simulink model "bh_model_crank_dynamics"  (R2022b)
settings: Solver=ode15s  StartTime=0.0  StopTime=45  RelTol=1e-4  AbsTol=1e-4  EnableMultiTasking=on
undefined symbols (not defined in the file): IC, params, sigbuilder_block, X, Y, Z
libraries: sm_lib x21, nesl_utility x19, simulink_extras x11, simulink x2
(part 1 of 2)
settings Model: Creator=bhorton  LastModifiedBy=bhorton
settings SolverCC: AutoScaleAbsTol=off  ZeroCrossAlgorithm=Adaptive  AlgebraicLoopSolver=TrustRegion
settings DataIOCC: LimitDataPoints=on  MaxDataPoints=10000
settings OptimizationCC: LifeSpan=inf
settings DebuggingCC: UnconnectedInputMsg=warning  UnconnectedOutputMsg=warning  UnconnectedLineMsg=warning  AllowSymbolicDim=off  SFUnexpectedBacktrackingDiag=warning  SFNoUnconditionalDefaultTransitionDiag=warning  SFExecutionAtInitializationDiag=none  SFMachineParentedDataDiag=warning  ArithmeticOperatorsInVariantConditions=warning
settings ModelReferenceCC: EnableRefExpFcnMdlSchedulingChecks=on
settings SFSimCC: SimUseLocalCustomCode=off  CustomCodeUndefinedFunction=UseInterfaceOnly
settings RTWCC: RTWUseLocalCustomCode=off  DLArmComputeVersion=19.05
settings CodeAppCC: StateflowObjectComments=on
settings GRTTargetCC: TargetLangStandard=C89/C90 (ANSI)
settings ConfigComp: CovMetricSettings=dw  CovSaveCumulativeToWorkspaceVar=on  CovSaveSingleToWorkspaceVar=on  CovExternalEMLEnable=off  CovSFcnEnable=off
settings SimscapeCC: SimscapeLogType=all  SimscapeLogSimulationStatistics=on  SimscapeLogToSDI=on  SimscapeLogLimitData=off  SimscapeLogDataHistory=10000
settings ExplorerConfigSet: InternalSimMechanicsExplorerSettings="<ExplorerConfiguration><canonicalview>default</canonicalview><AnimationSetting><BasePlaybackSpeed>1.0</BasePlaybackSpeed><PlaybackSpeedFactor>1.0</PlaybackSpeedFactor></AnimationSetting><TilePanel><TileInfo><Tiles Columns=\"1\" Count=\"1\" Rows=\"1\"><Column Weight=\"1\"/><Row Weight=\"1\"/><Tile Height=\"1\" Width=\"1\" X=\"0\" Y=\"0\"/></Tiles></TileInfo><SceneInfo><SceneViewer><BGColor><R>0.60000002384185791</R><G>0.60000002384185791</G><B>0.60000002384185791</B></BGColor><Camera><DoPerspective>off</DoPerspective><Position><X>0.384574720736644893</X><Y>0.1094227286849975</Y><Z>0.999999999924831462</Z></Position><Center><X>0.384574720736644893</X><Y>0.1094227286849975</Y><Z>-7.51685380606659237e-11</Z></Center><Up><X>0</X><Y>1</Y><Z>-0</Z></Up><ViewLimDist>1</ViewLimDist><YLim>0.563098594747124537</YLim><XLim>0.651675901785997991</XLim></Camera></SceneViewer></SceneInfo></TilePanel><MechEditorPanel><Cameras/><GfxPanelCameraMap/><VideoCreator><PlaybackSpeedRatio>1.0</PlaybackSpeedRatio><FrameRate>30</FrameRate><VideoFormat>Motion JPEG AVI</VideoFormat><FrameSize>auto</FrameSize></VideoCreator></MechEditorPanel></ExplorerConfiguration>"

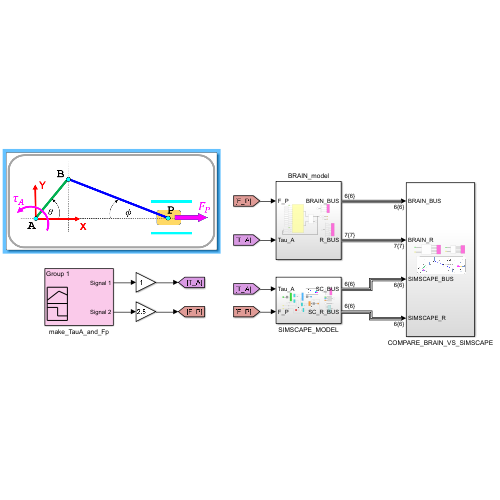
[thumbnail: Simulink's stored preview of the top-level diagram]
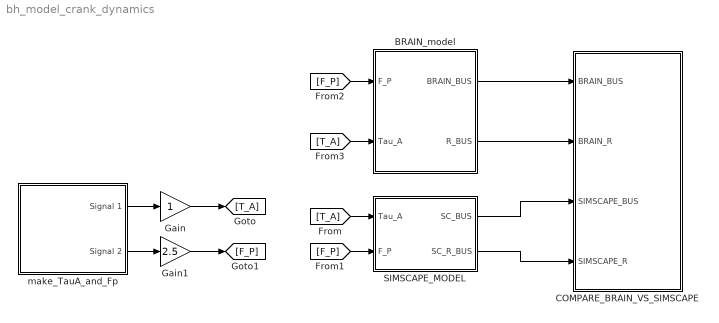
== system bh_model_crank_dynamics ==
  BRAIN_model : Subsystem
  COMPARE_BRAIN_VS_SIMSCAPE : Subsystem
  Gain : Gain
  Gain1 : Gain  Gain=2.5
  SIMSCAPE_MODEL : Subsystem
  make_TauA_and_Fp : Subsystem  Tag=STV Subsys  LoadFcn=sigbuilder_block('load');  StartFcn=sigbuilder_block('start');  StopFcn=sigbuilder_block('stop');  ClipboardFcn=sigbuilder_block('clipboard');  mask(Sigbuilder block){tuvar=[0:10]}
      mask help: Simulink:masks:SigbuilderBlock_MD
      mask init:
      | if ~strcmp(get_param(bdroot(gcbh),'SimulationStatus'),'stopped') tuvar = sigbuilder_block('maskInit'); end
      settings: CopyFcn=sigbuilder_block('copy');  DeleteFcn=sigbuilder_block('delete');  ModelCloseFcn=sigbuilder_block('modelClose');  PreSaveFcn=sigbuilder_block('preSave');  PauseFcn=sigbuilder_block('pause');  ContinueFcn=sigbuilder_block('continue');  NameChangeFcn=sigbuilder_block('namechange');  OpenFcn=sigbuilder_block('open',[883.5 110.25 550.5 258 ]);  CloseFcn=sigbuilder_block('close');
      mask Display: plot(0, 0, 100, 100,[2, 2, 32, 32, 2], [68, 8, 8, 68, 68],[32, 2], [38, 38], [32, 19, 2],[53, 60, 44], [32, 17, 17, 2],[16, 16, 31, 31]);txt = getActiveGroup(gcbh);text(2, 100, txt,'verticalAlignment', 'top');
  wires:
  make_TauA_and_Fp/1(Signal 1) -> Gain/1
  make_TauA_and_Fp/2(Signal 2) -> Gain1/1
  [T_A] -> SIMSCAPE_MODEL/1(Tau_A)
  [F_P] -> SIMSCAPE_MODEL/2(F_P)
  [F_P] -> BRAIN_model/1(F_P)
  [T_A] -> BRAIN_model/2(Tau_A)
  BRAIN_model/2(R_BUS) -> COMPARE_BRAIN_VS_SIMSCAPE/2(BRAIN_R)
  Gain/1 -> [T_A]
  Gain1/1 -> [F_P]
  BRAIN_model/1(BRAIN_BUS) -> COMPARE_BRAIN_VS_SIMSCAPE/1(BRAIN_BUS)
  SIMSCAPE_MODEL/1(SC_BUS) -> COMPARE_BRAIN_VS_SIMSCAPE/3(SIMSCAPE_BUS)
  SIMSCAPE_MODEL/2(SC_R_BUS) -> COMPARE_BRAIN_VS_SIMSCAPE/4(SIMSCAPE_R)

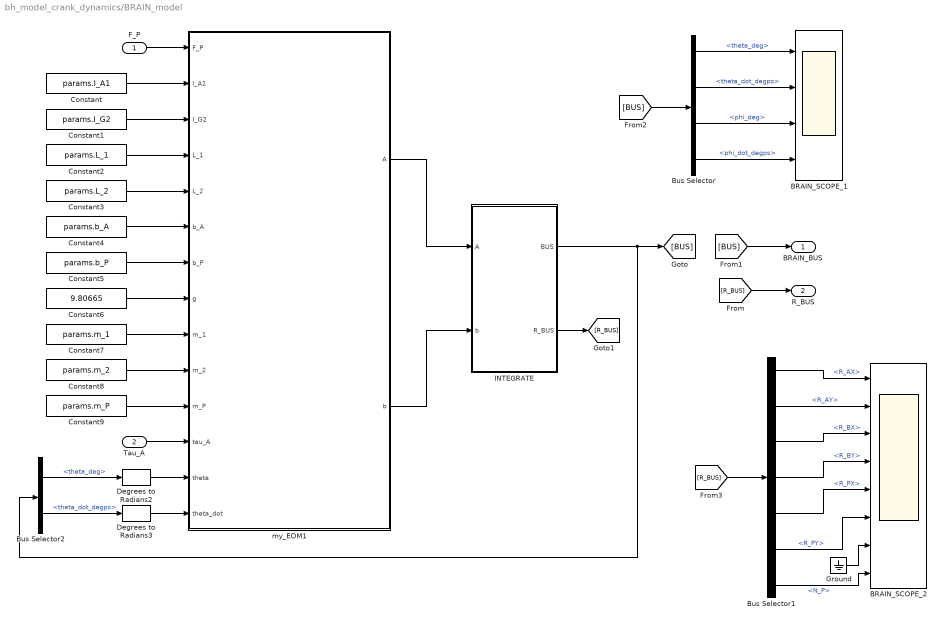
== system bh_model_crank_dynamics/BRAIN_model ==
  F_P : Inport
  Tau_A : Inport  Port=2
  BRAIN_SCOPE_1 : Scope  NumInputPorts=4
  BRAIN_SCOPE_2 : Scope  NumInputPorts=8
  Bus Selector : BusSelector  OutputSignals=theta_deg,theta_dot_degps,phi_deg,phi_dot_degps
  Bus Selector1 : BusSelector  OutputSignals=R_AX,R_AY,R_BX,R_BY,R_PX,R_PY,N_P
  Bus Selector2 : BusSelector  OutputSignals=theta_deg,theta_dot_degps
  Constant : Constant  Value=params.I_A1
  Constant1 : Constant  Value=params.I_G2
  Constant2 : Constant  Value=params.L_1
  Constant3 : Constant  Value=params.L_2
  Constant4 : Constant  Value=params.b_A
  Constant5 : Constant  Value=params.b_P
  Constant6 : Constant  Value=9.80665
  Constant7 : Constant  Value=params.m_1
  Constant8 : Constant  Value=params.m_2
  Constant9 : Constant  Value=params.m_P
  Degrees to Radians2 : simulink_extras/Transformations/Degrees to Radians
  Degrees to Radians3 : simulink_extras/Transformations/Degrees to Radians
  Ground : Ground
  INTEGRATE : Subsystem
  my_EOM1 : MATLAB Function  TreatAsAtomicUnit=on
  BRAIN_BUS : Outport
  R_BUS : Outport  Port=2
  wires:
  Bus Selector/2 -> BRAIN_SCOPE_1/2  "<theta_dot_degps>"
  Bus Selector/1 -> BRAIN_SCOPE_1/1  "<theta_deg>"
  Bus Selector/4 -> BRAIN_SCOPE_1/4  "<phi_dot_degps>"
  Bus Selector/3 -> BRAIN_SCOPE_1/3  "<phi_deg>"
  Bus Selector2/1 -> Degrees to Radians2/1  "<theta_deg>"
  Bus Selector2/2 -> Degrees to Radians3/1  "<theta_dot_degps>"
  F_P/1 -> my_EOM1/1(F_P)
  Constant/1 -> my_EOM1/2(I_A1)
  Constant1/1 -> my_EOM1/3(I_G2)
  Constant2/1 -> my_EOM1/4(L_1)
  Constant3/1 -> my_EOM1/5(L_2)
  Constant4/1 -> my_EOM1/6(b_A)
  Constant5/1 -> my_EOM1/7(b_P)
  Constant9/1 -> my_EOM1/11(m_P)
  Constant8/1 -> my_EOM1/10(m_2)
  Constant7/1 -> my_EOM1/9(m_1)
  Constant6/1 -> my_EOM1/8(g)
  Tau_A/1 -> my_EOM1/12(tau_A)
  Degrees to Radians2/1 -> my_EOM1/13(theta)
  Degrees to Radians3/1 -> my_EOM1/14(theta_dot)
  my_EOM1/1(A) -> INTEGRATE/1(A)
  my_EOM1/2(b) -> INTEGRATE/2(b)
  [BUS] -> Bus Selector/1
  [BUS] -> BRAIN_BUS/1
  [R_BUS] -> Bus Selector1/1
  Bus Selector1/1 -> BRAIN_SCOPE_2/1  "<R_AX>"
  Bus Selector1/2 -> BRAIN_SCOPE_2/2  "<R_AY>"
  Bus Selector1/3 -> BRAIN_SCOPE_2/3  "<R_BX>"
  Bus Selector1/4 -> BRAIN_SCOPE_2/4  "<R_BY>"
  Bus Selector1/5 -> BRAIN_SCOPE_2/5  "<R_PX>"
  Bus Selector1/6 -> BRAIN_SCOPE_2/6  "<R_PY>"
  Bus Selector1/7 -> BRAIN_SCOPE_2/8  "<N_P>"
  [R_BUS] -> R_BUS/1
  Ground/1 -> BRAIN_SCOPE_2/7
  INTEGRATE/1(BUS) -> Bus Selector2/1, [BUS]
  INTEGRATE/2(R_BUS) -> [R_BUS]

== system bh_model_crank_dynamics/COMPARE_BRAIN_VS_SIMSCAPE ==
  BRAIN_BUS : Inport
  BRAIN_R : Inport  Port=2
  SIMSCAPE_BUS : Inport  Port=3
  SIMSCAPE_R : Inport  Port=4
  SCOPE_POS_VEL_COMPARE : Scope  NumInputPorts=6
  SCOPE_REACTION_FORCES_COMPARE : Scope  NumInputPorts=6
  Subsystem : Subsystem
  Subsystem1 : Subsystem
  wires:
  BRAIN_BUS/1 -> Subsystem/1(BRAIN_BUS)
  SIMSCAPE_BUS/1 -> Subsystem/2(SIMSCAPE_BUS)
  Subsystem/1(theta_deg) -> SCOPE_POS_VEL_COMPARE/1
  Subsystem/2(theta_dot_degps) -> SCOPE_POS_VEL_COMPARE/2
  Subsystem/3(phi_deg) -> SCOPE_POS_VEL_COMPARE/3
  Subsystem/4(phi_dot_degps) -> SCOPE_POS_VEL_COMPARE/4
  Subsystem/5(P_pos) -> SCOPE_POS_VEL_COMPARE/5
  Subsystem/6(P_vel) -> SCOPE_POS_VEL_COMPARE/6
  Subsystem1/3(R_BX) -> SCOPE_REACTION_FORCES_COMPARE/3
  Subsystem1/4(R_BY) -> SCOPE_REACTION_FORCES_COMPARE/4
  Subsystem1/6(R_PY) -> SCOPE_REACTION_FORCES_COMPARE/6
  Subsystem1/2(R_AY) -> SCOPE_REACTION_FORCES_COMPARE/2
  Subsystem1/5(R_PX) -> SCOPE_REACTION_FORCES_COMPARE/5
  Subsystem1/1(R_AX) -> SCOPE_REACTION_FORCES_COMPARE/1
  BRAIN_R/1 -> Subsystem1/1(BRAIN_R)
  SIMSCAPE_R/1 -> Subsystem1/2(SIMSCAPE_R)

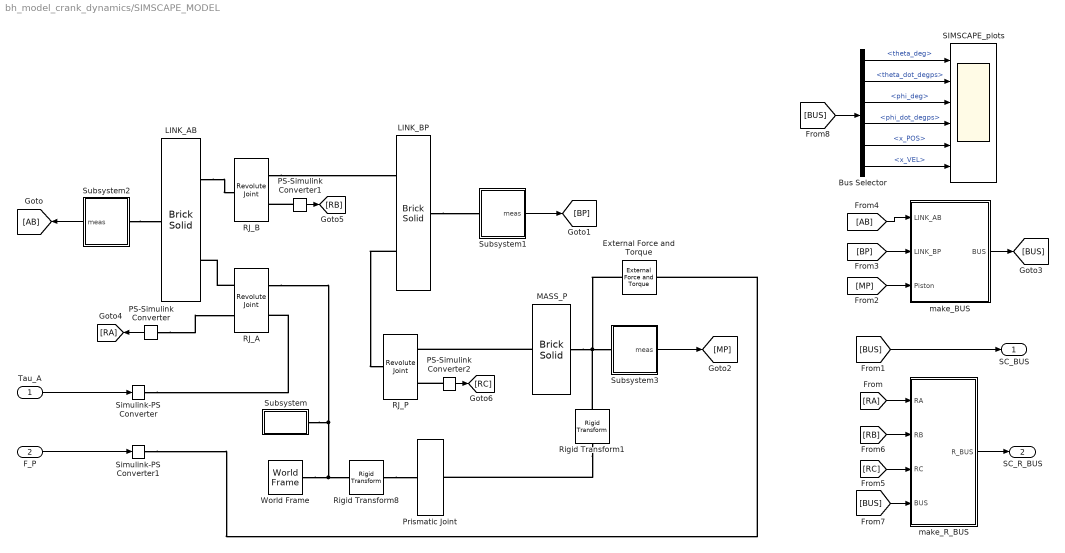
== system bh_model_crank_dynamics/SIMSCAPE_MODEL ==
  Tau_A : Inport
  F_P : Inport  Port=2
  Bus Selector : BusSelector  OutputSignals=theta_deg,theta_dot_degps,phi_deg,phi_dot_degps,x_POS,x_VEL
  External Force and Torque : sm_lib/Forces and Torques/External Force and Torque  ForceResolutionFrame=World  EnableForceX=on  EnableForceY=off  EnableForceZ=off  EnableForce=off  TorqueResolutionFrame=AttachedFrame  EnableTorqueX=off  EnableTorqueY=off  EnableTorqueZ=off  EnableTorque=off
  LINK_AB : sm_lib/Body Elements/Brick Solid  GraphicAmbientColor=[0.15 0.15 0.15 1.0]  BasedOnType=Density  BrickDimensions=params.L1_dims  BrickDimensionUnits=m  CenterOfMass=[0 0 0]  CenterOfMassUnits=m  GraphicDiffuseColor=[0.0 1.0 0.2]  Density=params.density  DensityUnits=kg/m^3  DoExposeReferenceFrame=on  GraphicEmissiveColor=[0.0 0.0 0.0 1.0]  ExportEntireGeometry=off  SerializedFrames=<Frames><Frame><Id>Frame1</Id><Value><Name>B</Name><Origin><Source>GeometricFeature</Source><FeatureName>+x surface</FeatureName></Origin><PrimaryAxis><DefinedDirection>+Z</DefinedDirection><Source>ReferenceFrame</Source><SourceDirection>+Z</SourceDirection><FeatureName></FeatureName></PrimaryAxis><SecondaryAxis><DefinedDirection>+X</DefinedDirection><Source>ReferenceFrame</Source><SourceDirection>+X</SourceDirection><FeatureName></FeatureName></SecondaryAxis></Value></Frame><Frame><Id>Frame2</Id><Value><Name>A</Name><Origin><Source>GeometricFeature</Source><FeatureName>-x surface</FeatureName></Origin><PrimaryAxis><DefinedDirection>+Z</DefinedDirection><Source>ReferenceFrame</Source><SourceDirection>+Z</SourceDirection><FeatureName></FeatureName></PrimaryAxis><SecondaryAxis><DefinedDirection>+X</DefinedDirection><Source>ReferenceFrame</Source><SourceDirection>+X</SourceDirection><FeatureName></FeatureName></SecondaryAxis></Value></Frame></Frames>  MarkerShape=Sphere  MarkerSize=10  GraphicType=FromGeometry  InertiaType=CalculateFromGeometry  Mass=1  MassUnits=kg  MomentsOfInertia=[1 1 1]  MomentsOfInertiaUnits=kg*m^2  GraphicOpacity=1.0  ProductsOfInertia=[0 0 0]  ProductsOfInertiaUnits=kg*m^2  GraphicShininess=75  GraphicSpecularColor=[0.5 0.5 0.5 1.0]  GraphicVisPropType=SimpleVisualProperties
  LINK_BP : sm_lib/Body Elements/Brick Solid  GraphicAmbientColor=[0.15 0.15 0.15 1.0]  BasedOnType=Density  BrickDimensions=params.L2_dims  BrickDimensionUnits=m  CenterOfMass=[0 0 0]  CenterOfMassUnits=m  GraphicDiffuseColor=[0.0 0.6 1.0]  Density=params.density  DensityUnits=kg/m^3  DoExposeReferenceFrame=on  GraphicEmissiveColor=[0.0 0.0 0.0 1.0]  ExportEntireGeometry=off  SerializedFrames=<Frames><Frame><Id>Frame1</Id><Value><Name>B</Name><Origin><Source>GeometricFeature</Source><FeatureName>-x surface</FeatureName></Origin><PrimaryAxis><DefinedDirection>+Z</DefinedDirection><Source>ReferenceFrame</Source><SourceDirection>+Z</SourceDirection><FeatureName></FeatureName></PrimaryAxis><SecondaryAxis><DefinedDirection>+X</DefinedDirection><Source>ReferenceFrame</Source><SourceDirection>+X</SourceDirection><FeatureName></FeatureName></SecondaryAxis></Value></Frame><Frame><Id>Frame2</Id><Value><Name>P</Name><Origin><Source>GeometricFeature</Source><FeatureName>+x surface</FeatureName></Origin><PrimaryAxis><DefinedDirection>+Z</DefinedDirection><Source>ReferenceFrame</Source><SourceDirection>+Z</SourceDirection><FeatureName></FeatureName></PrimaryAxis><SecondaryAxis><DefinedDirection>+X</DefinedDirection><Source>ReferenceFrame</Source><SourceDirection>+X</SourceDirection><FeatureName></FeatureName></SecondaryAxis></Value></Frame></Frames>  MarkerShape=Sphere  MarkerSize=10  GraphicType=FromGeometry  InertiaType=CalculateFromGeometry  Mass=1  MassUnits=kg  MomentsOfInertia=[1 1 1]  MomentsOfInertiaUnits=kg*m^2  GraphicOpacity=1.0  ProductsOfInertia=[0 0 0]  ProductsOfInertiaUnits=kg*m^2  GraphicShininess=75  GraphicSpecularColor=[0.5 0.5 0.5 1.0]  GraphicVisPropType=SimpleVisualProperties
  MASS_P : sm_lib/Body Elements/Brick Solid  GraphicAmbientColor=[0.15 0.15 0.15 1.0]  BasedOnType=Density  BrickDimensions=params.LP_dims  BrickDimensionUnits=m  CenterOfMass=[0 0 0]  CenterOfMassUnits=m  GraphicDiffuseColor=[1.0 0.6 0.2]  Density=params.density  DensityUnits=kg/m^3  DoExposeReferenceFrame=on  GraphicEmissiveColor=[0.0 0.0 0.0 1.0]  ExportEntireGeometry=off  SerializedFrames=<Frames><Frame><Id>Frame1</Id><Value><Name>B</Name><Origin><Source>CenterOfMassFrame</Source><FeatureName></FeatureName></Origin><PrimaryAxis><DefinedDirection>+Z</DefinedDirection><Source>ReferenceFrame</Source><SourceDirection>+Z</SourceDirection><FeatureName></FeatureName></PrimaryAxis><SecondaryAxis><DefinedDirection>+X</DefinedDirection><Source>ReferenceFrame</Source><SourceDirection>+X</SourceDirection><FeatureName></FeatureName></SecondaryAxis></Value></Frame></Frames>  MarkerShape=Sphere  MarkerSize=10  GraphicType=FromGeometry  InertiaType=CalculateFromGeometry  Mass=1  MassUnits=kg  MomentsOfInertia=[1 1 1]  MomentsOfInertiaUnits=kg*m^2  GraphicOpacity=1.0  ProductsOfInertia=[0 0 0]  ProductsOfInertiaUnits=kg*m^2  GraphicShininess=75  GraphicSpecularColor=[0.5 0.5 0.5 1.0]  GraphicVisPropType=SimpleVisualProperties
  PS-Simulink Converter : nesl_utility/PS-Simulink Converter  PhysicalDomain=network_engine_domain  SubClassName=ps_output  LeftPortType=input  RightPortType=output  PseudoPeriodic=off  Frequencies=[]  VectorFormat=1-D array  Unit=N  AffineConversion=off
  PS-Simulink Converter1 : nesl_utility/PS-Simulink Converter  PhysicalDomain=network_engine_domain  SubClassName=ps_output  LeftPortType=input  RightPortType=output  PseudoPeriodic=off  Frequencies=[]  VectorFormat=1-D array  Unit=N  AffineConversion=off
  PS-Simulink Converter2 : nesl_utility/PS-Simulink Converter  PhysicalDomain=network_engine_domain  SubClassName=ps_output  LeftPortType=input  RightPortType=output  PseudoPeriodic=off  Frequencies=[]  VectorFormat=1-D array  Unit=N  AffineConversion=off
  Prismatic Joint : sm_lib/Joints/Prismatic Joint  JointMode=Normal  SenseConstraintForce=off  SenseConstraintForceX=off  SenseConstraintForceY=off  SenseConstraintForceZ=off  SenseConstraintTorque=off  SenseConstraintTorqueX=off  SenseConstraintTorqueY=off  SenseConstraintTorqueZ=off  SenseTotalForce=off  SenseTotalForceX=off  SenseTotalForceY=off  SenseTotalForceZ=off  SenseTotalTorque=off  SenseTotalTorqueX=off  SenseTotalTorqueY=off  SenseTotalTorqueZ=off  CompositeWrenchDir=FollowerOnBase  CompositeWrenchFrame=BaseFrame  EquilibriumPosition=0  EquilibriumPositionUnits=m  SpringStiffness=0  SpringStiffnessUnits=N/m  DampingCoefficient=params.b_P  DampingCoefficientUnits=N/(m/s)  TorqueActuationMode=NoTorque  MotionActuationMode=ComputedMotion  SensePosition=off  SenseVelocity=off  SenseAcceleration=off  SenseTorqueForce=off  SenseLowerLimitTorqueForce=off  SenseUpperLimitTorqueForce=off  LowerLimitSpecify=off  LowerLimitBound=-1  LowerLimitBoundUnits=m  LowerLimitStiffness=1e6  LowerLimitStiffnessUnits=N/m  LowerLimitDamping=1e3  LowerLimitDampingUnits=N/(m/s)  LowerLimitTransitionRegionWidth=1e-4  LowerLimitTransitionRegionWidthUnits=m  UpperLimitSpecify=off  UpperLimitBound=1  UpperLimitBoundUnits=m  UpperLimitStiffness=1e6  UpperLimitStiffnessUnits=N/m  UpperLimitDamping=1e3  UpperLimitDampingUnits=N/(m/s)  UpperLimitTransitionRegionWidth=1e-4  UpperLimitTransitionRegionWidthUnits=m  PositionTargetSpecify=off  PositionTargetPriority=High  PositionTargetValue=0  PositionTargetValueUnits=m  VelocityTargetSpecify=off  VelocityTargetPriority=High  VelocityTargetValue=0  VelocityTargetValueUnits=m/s
  RJ_A : sm_lib/Joints/Revolute Joint  JointMode=Normal  SenseConstraintForce=on  SenseConstraintForceX=off  SenseConstraintForceY=off  SenseConstraintForceZ=off  SenseConstraintTorque=off  SenseConstraintTorqueX=off  SenseConstraintTorqueY=off  SenseConstraintTorqueZ=off  SenseTotalForce=off  SenseTotalForceX=off  SenseTotalForceY=off  SenseTotalForceZ=off  SenseTotalTorque=off  SenseTotalTorqueX=off  SenseTotalTorqueY=off  SenseTotalTorqueZ=off  CompositeWrenchDir=BaseOnFollower  CompositeWrenchFrame=BaseFrame  EquilibriumPosition=0  EquilibriumPositionUnits=deg  SpringStiffness=0  SpringStiffnessUnits=N*m/deg  DampingCoefficient=params.b_A  DampingCoefficientUnits=N*m/(rad/s)  TorqueActuationMode=InputTorque  MotionActuationMode=ComputedMotion  SensePosition=off  SenseVelocity=off  SenseAcceleration=off  SenseTorqueForce=off  SenseLowerLimitTorqueForce=off  SenseUpperLimitTorqueForce=off  LowerLimitSpecify=off  LowerLimitBound=-90  LowerLimitBoundUnits=deg  LowerLimitStiffness=1e4  LowerLimitStiffnessUnits=N*m/deg  LowerLimitDamping=10  LowerLimitDampingUnits=N*m/(deg/s)  LowerLimitTransitionRegionWidth=0.1  LowerLimitTransitionRegionWidthUnits=deg  UpperLimitSpecify=off  UpperLimitBound=90  UpperLimitBoundUnits=deg  UpperLimitStiffness=1e4  UpperLimitStiffnessUnits=N*m/deg  UpperLimitDamping=10  UpperLimitDampingUnits=N*m/(deg/s)  UpperLimitTransitionRegionWidth=0.1  UpperLimitTransitionRegionWidthUnits=deg  PositionTargetSpecify=on  PositionTargetPriority=High  PositionTargetValue=IC.theta_0  PositionTargetValueUnits=rad  VelocityTargetSpecify=on  VelocityTargetPriority=High  VelocityTargetValue=IC.theta_dot_0  VelocityTargetValueUnits=rad/s
  RJ_B : sm_lib/Joints/Revolute Joint  JointMode=Normal  SenseConstraintForce=on  SenseConstraintForceX=off  SenseConstraintForceY=off  SenseConstraintForceZ=off  SenseConstraintTorque=off  SenseConstraintTorqueX=off  SenseConstraintTorqueY=off  SenseConstraintTorqueZ=off  SenseTotalForce=off  SenseTotalForceX=off  SenseTotalForceY=off  SenseTotalForceZ=off  SenseTotalTorque=off  SenseTotalTorqueX=off  SenseTotalTorqueY=off  SenseTotalTorqueZ=off  CompositeWrenchDir=BaseOnFollower  CompositeWrenchFrame=FollowerFrame  EquilibriumPosition=0  EquilibriumPositionUnits=deg  SpringStiffness=0  SpringStiffnessUnits=N*m/deg  DampingCoefficient=0  DampingCoefficientUnits=N*m/(deg/s)  TorqueActuationMode=NoTorque  MotionActuationMode=ComputedMotion  SensePosition=off  SenseVelocity=off  SenseAcceleration=off  SenseTorqueForce=off  SenseLowerLimitTorqueForce=off  SenseUpperLimitTorqueForce=off  LowerLimitSpecify=off  LowerLimitBound=-90  LowerLimitBoundUnits=deg  LowerLimitStiffness=1e4  LowerLimitStiffnessUnits=N*m/deg  LowerLimitDamping=10  LowerLimitDampingUnits=N*m/(deg/s)  LowerLimitTransitionRegionWidth=0.1  LowerLimitTransitionRegionWidthUnits=deg  UpperLimitSpecify=off  UpperLimitBound=90  UpperLimitBoundUnits=deg  UpperLimitStiffness=1e4  UpperLimitStiffnessUnits=N*m/deg  UpperLimitDamping=10  UpperLimitDampingUnits=N*m/(deg/s)  UpperLimitTransitionRegionWidth=0.1  UpperLimitTransitionRegionWidthUnits=deg  PositionTargetSpecify=off  PositionTargetPriority=High  PositionTargetValue=0  PositionTargetValueUnits=rad  VelocityTargetSpecify=off  VelocityTargetPriority=High  VelocityTargetValue=0  VelocityTargetValueUnits=deg/s
  RJ_P : sm_lib/Joints/Revolute Joint  JointMode=Normal  SenseConstraintForce=on  SenseConstraintForceX=off  SenseConstraintForceY=off  SenseConstraintForceZ=off  SenseConstraintTorque=off  SenseConstraintTorqueX=off  SenseConstraintTorqueY=off  SenseConstraintTorqueZ=off  SenseTotalForce=off  SenseTotalForceX=off  SenseTotalForceY=off  SenseTotalForceZ=off  SenseTotalTorque=off  SenseTotalTorqueX=off  SenseTotalTorqueY=off  SenseTotalTorqueZ=off  CompositeWrenchDir=BaseOnFollower  CompositeWrenchFrame=FollowerFrame  EquilibriumPosition=0  EquilibriumPositionUnits=deg  SpringStiffness=0  SpringStiffnessUnits=N*m/deg  DampingCoefficient=0  DampingCoefficientUnits=N*m/(deg/s)  TorqueActuationMode=NoTorque  MotionActuationMode=ComputedMotion  SensePosition=off  SenseVelocity=off  SenseAcceleration=off  SenseTorqueForce=off  SenseLowerLimitTorqueForce=off  SenseUpperLimitTorqueForce=off  LowerLimitSpecify=off  LowerLimitBound=-90  LowerLimitBoundUnits=deg  LowerLimitStiffness=1e4  LowerLimitStiffnessUnits=N*m/deg  LowerLimitDamping=10  LowerLimitDampingUnits=N*m/(deg/s)  LowerLimitTransitionRegionWidth=0.1  LowerLimitTransitionRegionWidthUnits=deg  UpperLimitSpecify=off  UpperLimitBound=90  UpperLimitBoundUnits=deg  UpperLimitStiffness=1e4  UpperLimitStiffnessUnits=N*m/deg  UpperLimitDamping=10  UpperLimitDampingUnits=N*m/(deg/s)  UpperLimitTransitionRegionWidth=0.1  UpperLimitTransitionRegionWidthUnits=deg  PositionTargetSpecify=off  PositionTargetPriority=High  PositionTargetValue=0  PositionTargetValueUnits=rad  VelocityTargetSpecify=off  VelocityTargetPriority=High  VelocityTargetValue=0  VelocityTargetValueUnits=deg/s
  Rigid Transform1 : sm_lib/Frames and Transforms/Rigid Transform  TranslationMethod=None  TranslationStandardOffset=0  TranslationLengthUnit=m  TranslationStandardAxis=+Z  TranslationCartesianOffset=[0 0 0]  TranslationROffset=0  TranslationROffsetUnits=m  TranslationZOffset=0  TranslationZOffsetUnits=m  TranslationThetaOffset=0  TranslationThetaOffsetUnits=deg  RotationMethod=AlignedAxes  RotationAngleUnits=deg  RotationStandardAxis=+Z  RotationAngle=0.0  RotationArbitraryAxis=[0 0 1]  FollAlignAxisA=+Y  BaseAlignAxisA=+Y  FollAlignAxisB=+X  BaseAlignAxisB=+Z  RotationSequenceAxes=FollowerAxes  RotationSequence=XYX  RotationSequenceAngles=[0 0 0]  RotationSequenceAnglesUnits=deg  RotationMatrix=[1 0 0; 0 1 0; 0 0 1]  Quaternion=[1 0 0 0]
  Rigid Transform8 : sm_lib/Frames and Transforms/Rigid Transform  TranslationMethod=None  TranslationStandardOffset=0  TranslationLengthUnit=m  TranslationStandardAxis=+Z  TranslationCartesianOffset=[0 0 0]  TranslationROffset=0  TranslationROffsetUnits=m  TranslationZOffset=0  TranslationZOffsetUnits=m  TranslationThetaOffset=0  TranslationThetaOffsetUnits=deg  RotationMethod=AlignedAxes  RotationAngleUnits=deg  RotationStandardAxis=+Z  RotationAngle=0.0  RotationArbitraryAxis=[0 0 1]  FollAlignAxisA=+Y  BaseAlignAxisA=+Y  FollAlignAxisB=+Z  BaseAlignAxisB=+X  RotationSequenceAxes=FollowerAxes  RotationSequence=XYX  RotationSequenceAngles=[0 0 0]  RotationSequenceAnglesUnits=deg  RotationMatrix=[1 0 0; 0 1 0; 0 0 1]  Quaternion=[1 0 0 0]
  SIMSCAPE_plots : Scope  NumInputPorts=6
  Simulink-PS Converter : nesl_utility/Simulink-PS Converter  PhysicalDomain=network_engine_domain  SubClassName=ps_input  LeftPortType=input  RightPortType=output  PseudoPeriodic=off  Frequencies=[]  NoiseDistribution=none  NoiseParameters=[]  Unit=N*m  AffineConversion=off  FilteringAndDerivatives=provide  SimscapeFilterOrder=1  InputFilterTimeConstant=0.001  UdotUserProvided=0
  Simulink-PS Converter1 : nesl_utility/Simulink-PS Converter  PhysicalDomain=network_engine_domain  SubClassName=ps_input  LeftPortType=input  RightPortType=output  PseudoPeriodic=off  Frequencies=[]  NoiseDistribution=none  NoiseParameters=[]  Unit=N  AffineConversion=off  FilteringAndDerivatives=provide  SimscapeFilterOrder=1  InputFilterTimeConstant=0.001  UdotUserProvided=0
  Subsystem : Subsystem
  Subsystem1 : Subsystem
      mask Display: image('$imagefile'); % Use "Edit Image" on toolstrip to change.
  Subsystem2 : Subsystem
      mask Display: image('$imagefile'); % Use "Edit Image" on toolstrip to change.
  Subsystem3 : Subsystem
      mask Display: image('$imagefile'); % Use "Edit Image" on toolstrip to change.
  World Frame : sm_lib/Frames and Transforms/World Frame
  make_BUS : Subsystem
  make_R_BUS : Subsystem
  SC_BUS : Outport
  SC_R_BUS : Outport  Port=2
  wires:
  Bus Selector/1 -> SIMSCAPE_plots/1  "<theta_deg>"
  F_P/1 -> Simulink-PS Converter1/1
  Subsystem3/1(meas) -> [MP]
  Subsystem1/1(meas) -> [BP]
  [AB] -> make_BUS/1(LINK_AB)
  [MP] -> make_BUS/3(Piston)
  [BP] -> make_BUS/2(LINK_BP)
  Bus Selector/2 -> SIMSCAPE_plots/2  "<theta_dot_degps>"
  Tau_A/1 -> Simulink-PS Converter/1
  Bus Selector/3 -> SIMSCAPE_plots/3  "<phi_deg>"
  Bus Selector/5 -> SIMSCAPE_plots/5  "<x_POS>"
  Bus Selector/4 -> SIMSCAPE_plots/4  "<phi_dot_degps>"
  Bus Selector/6 -> SIMSCAPE_plots/6  "<x_VEL>"
  Subsystem2/1(meas) -> [AB]
  [BUS] -> SC_BUS/1
  PS-Simulink Converter/1 -> [RA]
  PS-Simulink Converter1/1 -> [RB]
  PS-Simulink Converter2/1 -> [RC]
  [RA] -> make_R_BUS/1(RA)
  [RB] -> make_R_BUS/2(RB)
  [RC] -> make_R_BUS/3(RC)
  make_R_BUS/1(R_BUS) -> SC_R_BUS/1
  [BUS] -> make_R_BUS/4(BUS)
  make_BUS/1(BUS) -> [BUS]
  [BUS] -> Bus Selector/1
  connections:
  LINK_BP/RConn1 -- Subsystem1/LConn1
  RJ_B/RConn1 -- LINK_BP/LConn1
  MASS_P/LConn1 -- RJ_P/RConn1
  Subsystem/LConn1 -- RJ_A/LConn1 -- World Frame/RConn1 -- Rigid Transform8/LConn1
  Simulink-PS Converter/RConn1 -- RJ_A/LConn2
  MASS_P/RConn1 -- External Force and Torque/RConn1 -- Rigid Transform1/RConn1 -- Subsystem3/LConn1
  Rigid Transform1/LConn1 -- Prismatic Joint/RConn1
  Rigid Transform8/RConn1 -- Prismatic Joint/LConn1
  Subsystem2/LConn1 -- LINK_AB/RConn1
  LINK_BP/LConn2 -- RJ_P/LConn1
  LINK_AB/LConn1 -- RJ_B/LConn1
  RJ_A/RConn1 -- LINK_AB/LConn2
  Simulink-PS Converter1/RConn1 -- External Force and Torque/LConn1
  PS-Simulink Converter1/LConn1 -- RJ_B/RConn2
  PS-Simulink Converter2/LConn1 -- RJ_P/RConn2
  PS-Simulink Converter/LConn1 -- RJ_A/RConn2

== system bh_model_crank_dynamics/make_TauA_and_Fp ==
  Demux : Demux  Tag=STV Demux  Outputs=2
      settings: DisplayOption=none
  FromWs : FromWorkspace  Tag=STV FromWs  VariableName=tuvar
      SigBuilderData=|
      | common.afterFinalStr = 'Extrapolate'
      | common.sampleTime = 0
      | dataSet.timeRange = [0 60]
      | dataSet.name = 'Group 1'
      | sbobj.Groups.Name = 'Group 1'
      | sbobj.Groups.Signals(1).Name = 'Signal 1'
      | sbobj.Groups.Signals(1).XData = [0 10 10 11 11 60]
      | sbobj.Groups.Signals(1).YData = [0 0 1 1 0 0]
      | sbobj.Groups.Signals(2).Name = 'Signal 2'
      | sbobj.Groups.Signals(2).XData = [0 25 25 27 27 60]
      | sbobj.Groups.Signals(2).YData = [0 0 1 1 0 0]
      | sbobj.Groups.TimeRange = [0 60]
  Signal 1 : Outport  Tag=STV Outport
  Signal 2 : Outport  Tag=STV Outport  Port=2
  wires:
  Demux/1 -> Signal 1/1
  FromWs/1 -> Demux/1
  Demux/2 -> Signal 2/1

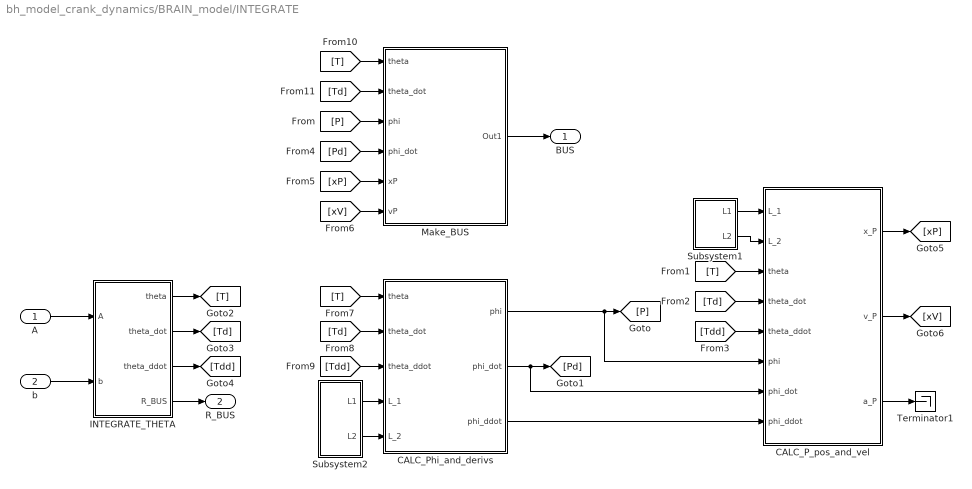
== system bh_model_crank_dynamics/BRAIN_model/INTEGRATE ==
  A : Inport
  b : Inport  Port=2
  CALC_P_pos_and_vel : MATLAB Function  TreatAsAtomicUnit=on
  CALC_Phi_and_derivs : MATLAB Function  TreatAsAtomicUnit=on
  INTEGRATE_THETA : Subsystem
  Make_BUS : Subsystem
  Subsystem1 : Subsystem
  Subsystem2 : Subsystem
  Terminator1 : Terminator
  BUS : Outport
  R_BUS : Outport  Port=2
  wires:
  A/1 -> INTEGRATE_THETA/1(A)
  b/1 -> INTEGRATE_THETA/2(b)
  CALC_P_pos_and_vel/2(v_P) -> [xV]
  CALC_P_pos_and_vel/1(x_P) -> [xP]
  CALC_P_pos_and_vel/3(a_P) -> Terminator1/1
  Subsystem2/1(L1) -> CALC_Phi_and_derivs/4(L_1)
  Subsystem2/2(L2) -> CALC_Phi_and_derivs/5(L_2)
  INTEGRATE_THETA/4(R_BUS) -> R_BUS/1
  Make_BUS/1(Out1) -> BUS/1
  CALC_Phi_and_derivs/1(phi) -> [P], CALC_P_pos_and_vel/6(phi)
  CALC_Phi_and_derivs/2(phi_dot) -> [Pd], CALC_P_pos_and_vel/7(phi_dot)
  CALC_Phi_and_derivs/3(phi_ddot) -> CALC_P_pos_and_vel/8(phi_ddot)
  Subsystem1/1(L1) -> CALC_P_pos_and_vel/1(L_1)
  Subsystem1/2(L2) -> CALC_P_pos_and_vel/2(L_2)
  [T] -> CALC_P_pos_and_vel/3(theta)
  [Tdd] -> CALC_P_pos_and_vel/5(theta_ddot)
  [Td] -> CALC_P_pos_and_vel/4(theta_dot)
  [P] -> Make_BUS/3(phi)
  [Pd] -> Make_BUS/4(phi_dot)
  [xP] -> Make_BUS/5(xP)
  [xV] -> Make_BUS/6(vP)
  INTEGRATE_THETA/1(theta) -> [T]
  INTEGRATE_THETA/2(theta_dot) -> [Td]
  INTEGRATE_THETA/3(theta_ddot) -> [Tdd]
  [T] -> CALC_Phi_and_derivs/1(theta)
  [Td] -> CALC_Phi_and_derivs/2(theta_dot)
  [Tdd] -> CALC_Phi_and_derivs/3(theta_ddot)
  [T] -> Make_BUS/1(theta)
  [Td] -> Make_BUS/2(theta_dot)

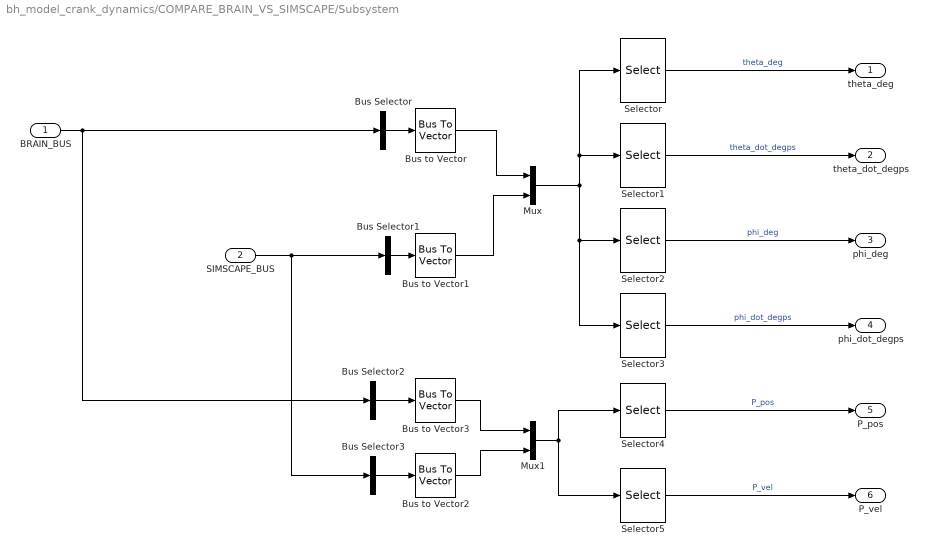
== system bh_model_crank_dynamics/COMPARE_BRAIN_VS_SIMSCAPE/Subsystem ==
  BRAIN_BUS : Inport
  SIMSCAPE_BUS : Inport  Port=2
  Bus Selector : BusSelector  OutputSignals=theta_deg,theta_dot_degps,phi_deg,phi_dot_degps  OutputAsBus=on
  Bus Selector1 : BusSelector  OutputSignals=theta_deg,theta_dot_degps,phi_deg,phi_dot_degps  OutputAsBus=on
  Bus Selector2 : BusSelector  OutputSignals=x_POS,x_VEL  OutputAsBus=on
  Bus Selector3 : BusSelector  OutputSignals=x_POS,x_VEL  OutputAsBus=on
  Bus to Vector{,1..3} (4 alike) : BusToVector
  Mux : Mux  Inputs=2
  Mux1 : Mux  Inputs=2
  Selector : Selector  InputPortWidth=8  IndexOptions=Index vector (dialog)  Indices=[1 5]  OutputSizes=1
  Selector1 : Selector  InputPortWidth=8  IndexOptions=Index vector (dialog)  Indices=[2 6]  OutputSizes=1
  Selector2 : Selector  InputPortWidth=8  IndexOptions=Index vector (dialog)  Indices=[3 7]  OutputSizes=1
  Selector3 : Selector  InputPortWidth=8  IndexOptions=Index vector (dialog)  Indices=[4 8]  OutputSizes=1
  Selector4 : Selector  InputPortWidth=4  IndexOptions=Index vector (dialog)  Indices=[1,3]  OutputSizes=1
  Selector5 : Selector  InputPortWidth=4  IndexOptions=Index vector (dialog)  Indices=[2,4]  OutputSizes=1
  theta_deg : Outport
  theta_dot_degps : Outport  Port=2
  phi_deg : Outport  Port=3
  phi_dot_degps : Outport  Port=4
  P_pos : Outport  Port=5
  P_vel : Outport  Port=6
  wires:
  Bus Selector/1 -> Bus to Vector/1
  Mux/1 -> Selector/1, Selector1/1, Selector3/1, Selector2/1
  Bus to Vector1/1 -> Mux/2
  Mux1/1 -> Selector5/1, Selector4/1
  Selector2/1 -> phi_deg/1  "phi_deg"
  Bus to Vector/1 -> Mux/1
  Bus Selector1/1 -> Bus to Vector1/1
  SIMSCAPE_BUS/1 -> Bus Selector3/1, Bus Selector1/1
  Bus Selector3/1 -> Bus to Vector2/1
  BRAIN_BUS/1 -> Bus Selector2/1, Bus Selector/1
  Bus to Vector3/1 -> Mux1/1
  Bus Selector2/1 -> Bus to Vector3/1
  Bus to Vector2/1 -> Mux1/2
  Selector5/1 -> P_vel/1  "P_vel"
  Selector3/1 -> phi_dot_degps/1  "phi_dot_degps"
  Selector/1 -> theta_deg/1  "theta_deg"
  Selector1/1 -> theta_dot_degps/1  "theta_dot_degps"
  Selector4/1 -> P_pos/1  "P_pos"

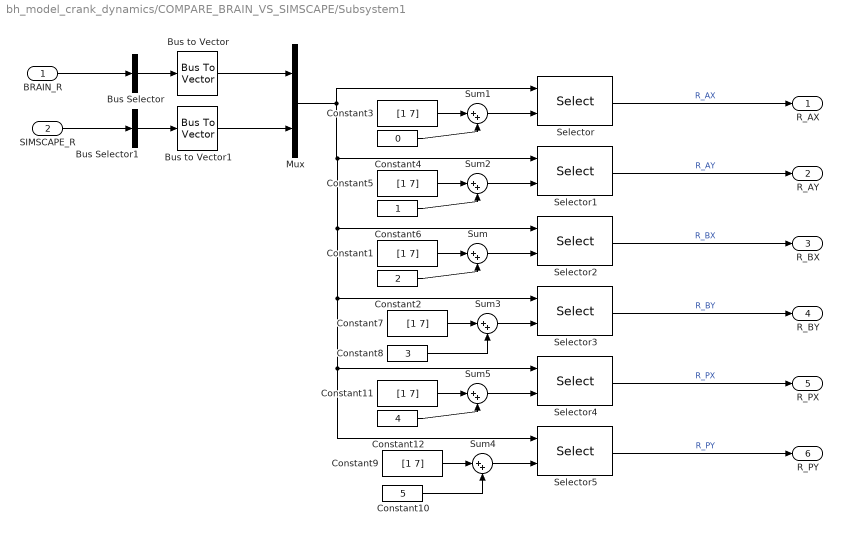
== system bh_model_crank_dynamics/COMPARE_BRAIN_VS_SIMSCAPE/Subsystem1 ==
  BRAIN_R : Inport
  SIMSCAPE_R : Inport  Port=2
  Bus Selector : BusSelector  OutputSignals=R_AX,R_AY,R_BX,R_BY,R_PX,R_PY  OutputAsBus=on
  Bus Selector1 : BusSelector  OutputSignals=R_AX,R_AY,R_BX,R_BY,R_PX,R_PY  OutputAsBus=on
  Bus to Vector : BusToVector
  Bus to Vector1 : BusToVector
  Constant{1,3,5,7,9,11} (6 alike) : Constant  Value=[1 7]
  Constant10 : Constant  Value=5
  Constant12 : Constant  Value=4
  Constant2 : Constant  Value=2
  Constant4 : Constant  Value=0
  Constant6 : Constant
  Constant8 : Constant  Value=3
  Mux : Mux  Inputs=2
  Selector{,1..5} (6 alike) : Selector  InputPortWidth=12  IndexOptions=Index vector (port)  Indices=[1 5]  OutputSizes=1
  Sum{,1..5} (6 alike) : Sum  Inputs=|++
  R_AX : Outport
  R_AY : Outport  Port=2
  R_BX : Outport  Port=3
  R_BY : Outport  Port=4
  R_PX : Outport  Port=5
  R_PY : Outport  Port=6
  wires:
  Mux/1 -> Selector/1, Selector2/1, Selector3/1, Selector4/1, Selector5/1, Selector1/1
  Selector2/1 -> R_BX/1  "R_BX"
  Constant10/1 -> Sum4/2
  Bus Selector1/1 -> Bus to Vector1/1
  Constant12/1 -> Sum5/2
  Constant3/1 -> Sum1/1
  Sum5/1 -> Selector4/2
  Constant5/1 -> Sum2/1
  Bus Selector/1 -> Bus to Vector/1
  Sum3/1 -> Selector3/2
  Selector1/1 -> R_AY/1  "R_AY"
  Bus to Vector1/1 -> Mux/2
  Constant11/1 -> Sum5/1
  Constant2/1 -> Sum/2
  Sum1/1 -> Selector/2
  Sum4/1 -> Selector5/2
  Constant4/1 -> Sum1/2
  Constant1/1 -> Sum/1
  Sum2/1 -> Selector1/2
  Constant8/1 -> Sum3/2
  Sum/1 -> Selector2/2
  Bus to Vector/1 -> Mux/1
  Constant7/1 -> Sum3/1
  Constant6/1 -> Sum2/2
  Constant9/1 -> Sum4/1
  Selector4/1 -> R_PX/1  "R_PX"
  Selector/1 -> R_AX/1  "R_AX"
  Selector5/1 -> R_PY/1  "R_PY"
  Selector3/1 -> R_BY/1  "R_BY"
  SIMSCAPE_R/1 -> Bus Selector1/1
  BRAIN_R/1 -> Bus Selector/1

== system bh_model_crank_dynamics/SIMSCAPE_MODEL/Subsystem ==
  Graphic : sm_lib/Body Elements/Graphic  GraphicType=Marker  MarkerShape=Frame  MarkerSize=36  GraphicVisPropType=SimpleVisualProperties  GraphicDiffuseColor=[0.0 0.0 0.0]  GraphicSpecularColor=[0.5 0.5 0.5 1.0]  GraphicAmbientColor=[0.15 0.15 0.15 1.0]  GraphicEmissiveColor=[0.0 0.0 0.0 1.0]  GraphicShininess=75  GraphicOpacity=1.0
  Mechanism Configuration : sm_lib/Utilities/Mechanism Configuration  UniformGravity=Constant  GravityVector=[0, -9.80665, 0]  GravityUnits=m/s^2  LinearizationDelta=0.001  JointModeTransitionNonlinearIterations=2
  Solver Configuration : nesl_utility/Solver Configuration  PhysicalDomain=network_engine_domain  SubClassName=solver  LeftPortType=input  RightPortType=generic  Tones=[]  Harmonics=[]  SimulateNoise=off  Profile=off  UseLocalSampling=off  EnableSwitchedLinearOptims=on  FrequencyDomain=off  UseCCode=off  RelTol=0.001  AbsTol=1e-06  MinStep=1e-09  ToWorkspace=off  RevertToSquareIcSolve=off  NumHomotopyIterations=100  PhasorMode=off  PhasorModeNumHarmonics=1  ConsistencySolver=NEWTON_FTOL  IndexReductionMethod=DerivativeReplacement  DoDC=off  ResidualTolerance=1e-09  ConsistencyTolSource=GLOBAL  ConsistencyAbsTol=0.001  ConsistencyRelTol=0.001  ConsistencyTolFactor=0.001  UseLocalSolver=off  LocalSolverChoice=NE_BACKWARD_EULER_ADVANCER  ResolveIndetEquations=on  FunctionEvalNumThread=1  LocalSolverSampleTime=0.001  DoFixedCost=off  MaxNonlinIter=3  MaxModeIter=2  ComputeImpulses=off  ImpulseIterations=2  LinearAlgebra=Sparse  LinearAlgebraNumThread=0  EquationFormulation=NE_TIME_EF  DelaysMemoryBudget=1024  AutomaticFiltering=on  FilteringTimeConstant=0.001  PartitionStorageMethod=AS_NEEDED  PartitionMemoryBudget=1024  PartitionMethod=FAST
  Mechanism Configuration1 : PMIOPort  Side=Left
  connections:
  Solver Configuration/RConn1 -- Mechanism Configuration/RConn1 -- Graphic/RConn1 -- Mechanism Configuration1/RConn1

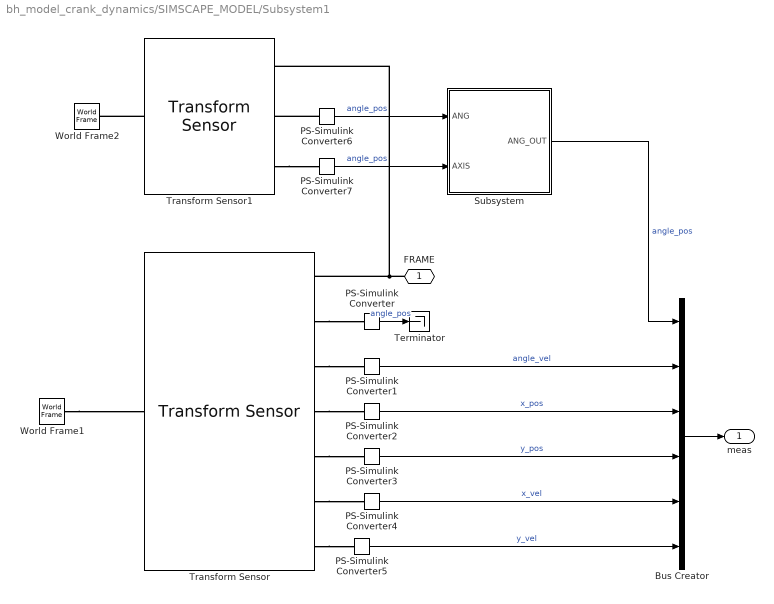
== system bh_model_crank_dynamics/SIMSCAPE_MODEL/Subsystem1 ==
  Bus Creator : BusCreator  Inputs=6
  PS-Simulink Converter : nesl_utility/PS-Simulink Converter  PhysicalDomain=network_engine_domain  SubClassName=ps_output  LeftPortType=input  RightPortType=output  PseudoPeriodic=off  Frequencies=[]  VectorFormat=1-D array  Unit=rad  AffineConversion=off
  PS-Simulink Converter1 : nesl_utility/PS-Simulink Converter  PhysicalDomain=network_engine_domain  SubClassName=ps_output  LeftPortType=input  RightPortType=output  PseudoPeriodic=off  Frequencies=[]  VectorFormat=1-D array  Unit=rad/s  AffineConversion=off
  PS-Simulink Converter2 : nesl_utility/PS-Simulink Converter  PhysicalDomain=network_engine_domain  SubClassName=ps_output  LeftPortType=input  RightPortType=output  PseudoPeriodic=off  Frequencies=[]  VectorFormat=1-D array  Unit=m  AffineConversion=on
  PS-Simulink Converter3 : nesl_utility/PS-Simulink Converter  PhysicalDomain=network_engine_domain  SubClassName=ps_output  LeftPortType=input  RightPortType=output  PseudoPeriodic=off  Frequencies=[]  VectorFormat=1-D array  Unit=m  AffineConversion=on
  PS-Simulink Converter4 : nesl_utility/PS-Simulink Converter  PhysicalDomain=network_engine_domain  SubClassName=ps_output  LeftPortType=input  RightPortType=output  PseudoPeriodic=off  Frequencies=[]  VectorFormat=1-D array  Unit=m/s  AffineConversion=on
  PS-Simulink Converter5 : nesl_utility/PS-Simulink Converter  PhysicalDomain=network_engine_domain  SubClassName=ps_output  LeftPortType=input  RightPortType=output  PseudoPeriodic=off  Frequencies=[]  VectorFormat=1-D array  Unit=m/s  AffineConversion=on
  PS-Simulink Converter6 : nesl_utility/PS-Simulink Converter  PhysicalDomain=network_engine_domain  SubClassName=ps_output  LeftPortType=input  RightPortType=output  PseudoPeriodic=off  Frequencies=[]  VectorFormat=1-D array  Unit=rad  AffineConversion=off
  PS-Simulink Converter7 : nesl_utility/PS-Simulink Converter  PhysicalDomain=network_engine_domain  SubClassName=ps_output  LeftPortType=input  RightPortType=output  PseudoPeriodic=off  Frequencies=[]  VectorFormat=1-D array  Unit=1  AffineConversion=off
  Subsystem : Subsystem
  Terminator : Terminator
  Transform Sensor : sm_lib/Frames and Transforms/Transform Sensor  MeasurementFrame=World  SenseAngle=on  SenseAxis=off  SenseQ=off  SenseR=off  SenseRotationSequence=off  RotationSequence=XYX  SenseOmegaX=off  SenseOmegaY=off  SenseOmegaZ=on  SenseQDot=off  SenseRDot=off  SenseAlphaX=off  SenseAlphaY=off  SenseAlphaZ=off  SenseQDDot=off  SenseRDDot=off  SenseX=on  SenseY=on  SenseZ=off  SenseRad=off  SenseAzim=off  SenseDist=off  SenseInc=off  SenseXDot=on  SenseYDot=on  SenseZDot=off  SenseRadDot=off  SenseAzimDot=off  SenseDistDot=off  SenseIncDot=off  SenseXDDot=off  SenseYDDot=off  SenseZDDot=off  SenseRadDDot=off  SenseAzimDDot=off  SenseDistDDot=off  SenseIncDDot=off
  Transform Sensor1 : sm_lib/Frames and Transforms/Transform Sensor  MeasurementFrame=World  SenseAngle=on  SenseAxis=on  SenseQ=off  SenseR=off  SenseRotationSequence=off  RotationSequence=XYX  SenseOmegaX=off  SenseOmegaY=off  SenseOmegaZ=off  SenseQDot=off  SenseRDot=off  SenseAlphaX=off  SenseAlphaY=off  SenseAlphaZ=off  SenseQDDot=off  SenseRDDot=off  SenseX=off  SenseY=off  SenseZ=off  SenseRad=off  SenseAzim=off  SenseDist=off  SenseInc=off  SenseXDot=off  SenseYDot=off  SenseZDot=off  SenseRadDot=off  SenseAzimDot=off  SenseDistDot=off  SenseIncDot=off  SenseXDDot=off  SenseYDDot=off  SenseZDDot=off  SenseRadDDot=off  SenseAzimDDot=off  SenseDistDDot=off  SenseIncDDot=off
  World Frame1 : sm_lib/Frames and Transforms/World Frame
  World Frame2 : sm_lib/Frames and Transforms/World Frame
  FRAME : PMIOPort  Side=Left
  meas : Outport
  wires:
  PS-Simulink Converter1/1 -> Bus Creator/2  "angle_vel"
  PS-Simulink Converter2/1 -> Bus Creator/3  "x_pos"
  PS-Simulink Converter3/1 -> Bus Creator/4  "y_pos"
  Bus Creator/1 -> meas/1
  PS-Simulink Converter4/1 -> Bus Creator/5  "x_vel"
  PS-Simulink Converter5/1 -> Bus Creator/6  "y_vel"
  PS-Simulink Converter6/1 -> Subsystem/1(ANG)  "angle_pos"
  PS-Simulink Converter7/1 -> Subsystem/2(AXIS)  "angle_pos"
  PS-Simulink Converter/1 -> Terminator/1  "angle_pos"
  Subsystem/1(ANG_OUT) -> Bus Creator/1  "angle_pos"
  connections:
  Transform Sensor/RConn1 -- FRAME/RConn1 -- Transform Sensor1/RConn1
  World Frame1/RConn1 -- Transform Sensor/LConn1
  Transform Sensor/RConn2 -- PS-Simulink Converter/LConn1
  Transform Sensor/RConn3 -- PS-Simulink Converter1/LConn1
  Transform Sensor/RConn4 -- PS-Simulink Converter2/LConn1
  Transform Sensor/RConn5 -- PS-Simulink Converter3/LConn1
  Transform Sensor/RConn6 -- PS-Simulink Converter4/LConn1
  Transform Sensor/RConn7 -- PS-Simulink Converter5/LConn1
  Transform Sensor1/LConn1 -- World Frame2/RConn1
  PS-Simulink Converter6/LConn1 -- Transform Sensor1/RConn2
  Transform Sensor1/RConn3 -- PS-Simulink Converter7/LConn1

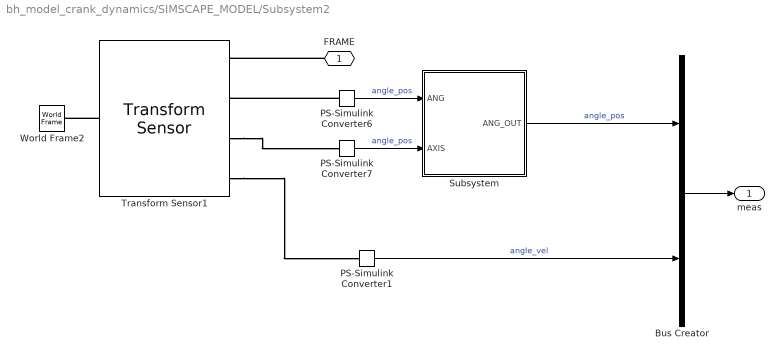
== system bh_model_crank_dynamics/SIMSCAPE_MODEL/Subsystem2 ==
  Bus Creator : BusCreator  Inputs=2
  PS-Simulink Converter1 : nesl_utility/PS-Simulink Converter  PhysicalDomain=network_engine_domain  SubClassName=ps_output  LeftPortType=input  RightPortType=output  PseudoPeriodic=off  Frequencies=[]  VectorFormat=1-D array  Unit=rad/s  AffineConversion=off
  PS-Simulink Converter6 : nesl_utility/PS-Simulink Converter  PhysicalDomain=network_engine_domain  SubClassName=ps_output  LeftPortType=input  RightPortType=output  PseudoPeriodic=off  Frequencies=[]  VectorFormat=1-D array  Unit=rad  AffineConversion=off
  PS-Simulink Converter7 : nesl_utility/PS-Simulink Converter  PhysicalDomain=network_engine_domain  SubClassName=ps_output  LeftPortType=input  RightPortType=output  PseudoPeriodic=off  Frequencies=[]  VectorFormat=1-D array  Unit=1  AffineConversion=off
  Subsystem : Subsystem
  Transform Sensor1 : sm_lib/Frames and Transforms/Transform Sensor  MeasurementFrame=World  SenseAngle=on  SenseAxis=on  SenseQ=off  SenseR=off  SenseRotationSequence=off  RotationSequence=XYX  SenseOmegaX=off  SenseOmegaY=off  SenseOmegaZ=on  SenseQDot=off  SenseRDot=off  SenseAlphaX=off  SenseAlphaY=off  SenseAlphaZ=off  SenseQDDot=off  SenseRDDot=off  SenseX=off  SenseY=off  SenseZ=off  SenseRad=off  SenseAzim=off  SenseDist=off  SenseInc=off  SenseXDot=off  SenseYDot=off  SenseZDot=off  SenseRadDot=off  SenseAzimDot=off  SenseDistDot=off  SenseIncDot=off  SenseXDDot=off  SenseYDDot=off  SenseZDDot=off  SenseRadDDot=off  SenseAzimDDot=off  SenseDistDDot=off  SenseIncDDot=off
  World Frame2 : sm_lib/Frames and Transforms/World Frame
  FRAME : PMIOPort  Side=Left
  meas : Outport
  wires:
  PS-Simulink Converter1/1 -> Bus Creator/2  "angle_vel"
  Bus Creator/1 -> meas/1
  PS-Simulink Converter6/1 -> Subsystem/1(ANG)  "angle_pos"
  PS-Simulink Converter7/1 -> Subsystem/2(AXIS)  "angle_pos"
  Subsystem/1(ANG_OUT) -> Bus Creator/1  "angle_pos"
  connections:
  FRAME/RConn1 -- Transform Sensor1/RConn1
  Transform Sensor1/RConn4 -- PS-Simulink Converter1/LConn1
  Transform Sensor1/LConn1 -- World Frame2/RConn1
  PS-Simulink Converter6/LConn1 -- Transform Sensor1/RConn2
  Transform Sensor1/RConn3 -- PS-Simulink Converter7/LConn1

== system bh_model_crank_dynamics/SIMSCAPE_MODEL/Subsystem3 ==
  Bus Creator : BusCreator  Inputs=2
  PS-Simulink Converter2 : nesl_utility/PS-Simulink Converter  PhysicalDomain=network_engine_domain  SubClassName=ps_output  LeftPortType=input  RightPortType=output  PseudoPeriodic=off  Frequencies=[]  VectorFormat=1-D array  Unit=m  AffineConversion=on
  PS-Simulink Converter4 : nesl_utility/PS-Simulink Converter  PhysicalDomain=network_engine_domain  SubClassName=ps_output  LeftPortType=input  RightPortType=output  PseudoPeriodic=off  Frequencies=[]  VectorFormat=1-D array  Unit=m/s  AffineConversion=on
  Transform Sensor : sm_lib/Frames and Transforms/Transform Sensor  MeasurementFrame=World  SenseAngle=off  SenseAxis=off  SenseQ=off  SenseR=off  SenseRotationSequence=off  RotationSequence=XYX  SenseOmegaX=off  SenseOmegaY=off  SenseOmegaZ=off  SenseQDot=off  SenseRDot=off  SenseAlphaX=off  SenseAlphaY=off  SenseAlphaZ=off  SenseQDDot=off  SenseRDDot=off  SenseX=on  SenseY=off  SenseZ=off  SenseRad=off  SenseAzim=off  SenseDist=off  SenseInc=off  SenseXDot=on  SenseYDot=off  SenseZDot=off  SenseRadDot=off  SenseAzimDot=off  SenseDistDot=off  SenseIncDot=off  SenseXDDot=off  SenseYDDot=off  SenseZDDot=off  SenseRadDDot=off  SenseAzimDDot=off  SenseDistDDot=off  SenseIncDDot=off
  World Frame1 : sm_lib/Frames and Transforms/World Frame
  MP : PMIOPort  Side=Left
  meas : Outport
  wires:
  PS-Simulink Converter2/1 -> Bus Creator/1  "x_pos"
  Bus Creator/1 -> meas/1
  PS-Simulink Converter4/1 -> Bus Creator/2  "x_vel"
  connections:
  World Frame1/RConn1 -- Transform Sensor/LConn1
  Transform Sensor/RConn3 -- PS-Simulink Converter4/LConn1
  Transform Sensor/RConn2 -- PS-Simulink Converter2/LConn1
  Transform Sensor/RConn1 -- MP/RConn1

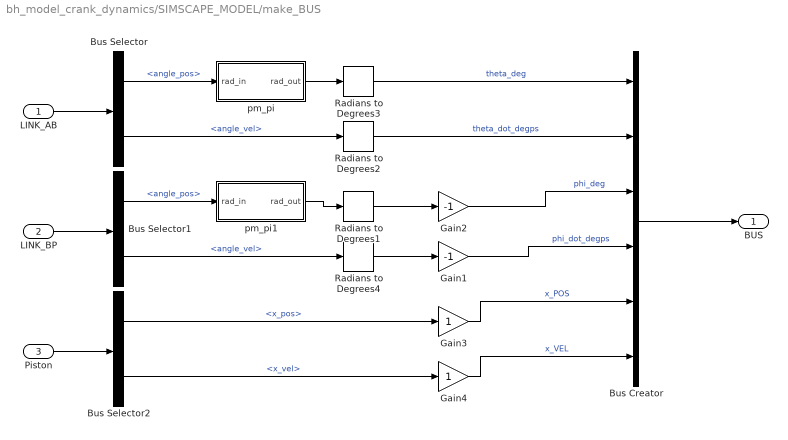
== system bh_model_crank_dynamics/SIMSCAPE_MODEL/make_BUS ==
  LINK_AB : Inport
  LINK_BP : Inport  Port=2
  Piston : Inport  Port=3
  Bus Creator : BusCreator  Inputs=6
  Bus Selector : BusSelector  OutputSignals=angle_pos,angle_vel
  Bus Selector1 : BusSelector  OutputSignals=angle_pos,angle_vel
  Bus Selector2 : BusSelector  OutputSignals=x_pos,x_vel
  Gain1 : Gain  Gain=-1
  Gain2 : Gain  Gain=-1
  Gain3 : Gain
  Gain4 : Gain
  Radians to Degrees{1..4} (4 alike) : simulink_extras/Transformations/Radians to Degrees
  pm_pi : Subsystem
  pm_pi1 : Subsystem
  BUS : Outport
  wires:
  Bus Selector1/2 -> Radians to Degrees4/1  "<angle_vel>"
  LINK_BP/1 -> Bus Selector1/1
  Radians to Degrees2/1 -> Bus Creator/2  "theta_dot_degps"
  LINK_AB/1 -> Bus Selector/1
  Radians to Degrees3/1 -> Bus Creator/1  "theta_deg"
  Bus Selector/2 -> Radians to Degrees2/1  "<angle_vel>"
  Bus Selector1/1 -> pm_pi1/1(rad_in)  "<angle_pos>"
  Gain2/1 -> Bus Creator/3  "phi_deg"
  Bus Creator/1 -> BUS/1
  Piston/1 -> Bus Selector2/1
  Bus Selector2/1 -> Gain3/1  "<x_pos>"
  Gain3/1 -> Bus Creator/5  "x_POS"
  Bus Selector2/2 -> Gain4/1  "<x_vel>"
  Gain4/1 -> Bus Creator/6  "x_VEL"
  Gain1/1 -> Bus Creator/4  "phi_dot_degps"
  Bus Selector/1 -> pm_pi/1(rad_in)  "<angle_pos>"
  pm_pi/1(rad_out) -> Radians to Degrees3/1
  pm_pi1/1(rad_out) -> Radians to Degrees1/1
  Radians to Degrees1/1 -> Gain2/1
  Radians to Degrees4/1 -> Gain1/1

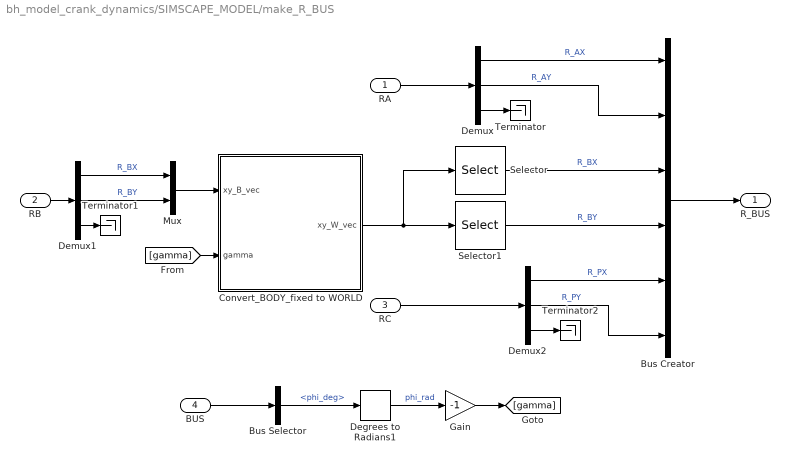
== system bh_model_crank_dynamics/SIMSCAPE_MODEL/make_R_BUS ==
  RA : Inport
  RB : Inport  Port=2
  RC : Inport  Port=3
  BUS : Inport  Port=4
  Bus Creator : BusCreator  Inputs=6
  Bus Selector : BusSelector  OutputSignals=phi_deg
  Convert_BODY_fixed to WORLD : MATLAB Function  TreatAsAtomicUnit=on
  Degrees to Radians1 : simulink_extras/Transformations/Degrees to Radians
  Demux : Demux  Outputs=3
  Demux1 : Demux  Outputs=3
  Demux2 : Demux  Outputs=3
  Gain : Gain  Gain=-1
  Mux : Mux  Inputs=2
  Selector : Selector  InputPortWidth=2  IndexOptions=Index vector (dialog)  Indices=1  OutputSizes=1
  Selector1 : Selector  InputPortWidth=2  IndexOptions=Index vector (dialog)  Indices=2  OutputSizes=1
  Terminator : Terminator
  Terminator1 : Terminator
  Terminator2 : Terminator
  R_BUS : Outport
  wires:
  RA/1 -> Demux/1
  Bus Creator/1 -> R_BUS/1
  Demux/3 -> Terminator/1
  Demux2/3 -> Terminator2/1
  Demux/1 -> Bus Creator/1  "R_AX"
  Demux/2 -> Bus Creator/2  "R_AY"
  Selector/1 -> Bus Creator/3  "R_BX"
  Demux2/1 -> Bus Creator/5  "R_PX"
  Demux2/2 -> Bus Creator/6  "R_PY"
  RC/1 -> Demux2/1
  Gain/1 -> [gamma]
  Bus Selector/1 -> Degrees to Radians1/1  "<phi_deg>"
  BUS/1 -> Bus Selector/1
  Degrees to Radians1/1 -> Gain/1  "phi_rad"
  Convert_BODY_fixed to WORLD/1(xy_W_vec) -> Selector1/1, Selector/1
  Mux/1 -> Convert_BODY_fixed to WORLD/1(xy_B_vec)
  Demux1/3 -> Terminator1/1
  RB/1 -> Demux1/1
  Demux1/1 -> Mux/1  "R_BX"
  Demux1/2 -> Mux/2  "R_BY"
  [gamma] -> Convert_BODY_fixed to WORLD/2(gamma)
  Selector1/1 -> Bus Creator/4  "R_BY"

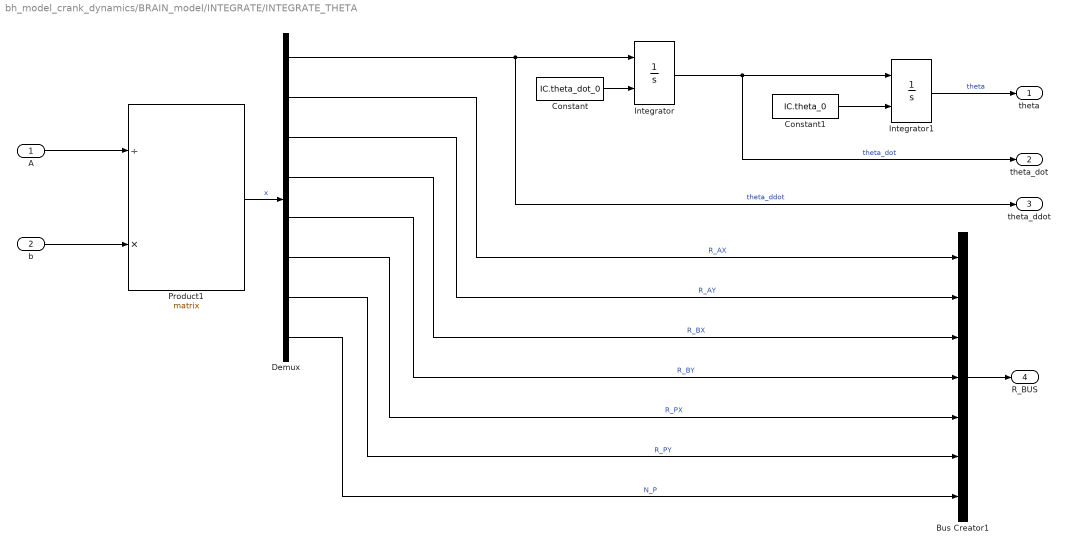
== system bh_model_crank_dynamics/BRAIN_model/INTEGRATE/INTEGRATE_THETA ==
  A : Inport
  b : Inport  Port=2
  Bus Creator1 : BusCreator  Inputs=7
  Constant : Constant  Value=IC.theta_dot_0
  Constant1 : Constant  Value=IC.theta_0
  Demux : Demux  Outputs=8
  Integrator : Integrator  InitialConditionSource=external
  Integrator1 : Integrator  InitialConditionSource=external  WrapState=on
  Product1 : Product  Inputs=/*  Multiplication=Matrix(*)
  theta : Outport
  theta_dot : Outport  Port=2
  theta_ddot : Outport  Port=3
  R_BUS : Outport  Port=4
  wires:
  A/1 -> Product1/1
  b/1 -> Product1/2
  Integrator1/1 -> theta/1  "theta"
  Constant/1 -> Integrator/2
  Constant1/1 -> Integrator1/2
  Integrator/1 -> theta_dot/1, Integrator1/1  "theta_dot"
  Product1/1 -> Demux/1  "x"
  Demux/8 -> Bus Creator1/7  "N_P"
  Demux/7 -> Bus Creator1/6  "R_PY"
  Demux/6 -> Bus Creator1/5  "R_PX"
  Demux/5 -> Bus Creator1/4  "R_BY"
  Demux/4 -> Bus Creator1/3  "R_BX"
  Demux/3 -> Bus Creator1/2  "R_AY"
  Demux/2 -> Bus Creator1/1  "R_AX"
  Bus Creator1/1 -> R_BUS/1
  Demux/1 -> theta_ddot/1, Integrator/1  "theta_ddot"

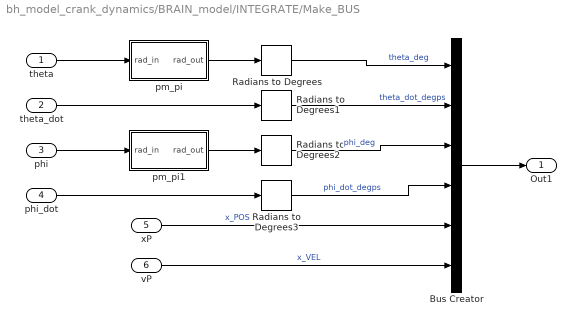
== system bh_model_crank_dynamics/BRAIN_model/INTEGRATE/Make_BUS ==
  theta : Inport
  theta_dot : Inport  Port=2
  phi : Inport  Port=3
  phi_dot : Inport  Port=4
  xP : Inport  Port=5
  vP : Inport  Port=6
  Bus Creator : BusCreator  Inputs=6
  Radians to Degrees{,1..3} (4 alike) : simulink_extras/Transformations/Radians to Degrees
  pm_pi : Subsystem
  pm_pi1 : Subsystem
  Out1 : Outport
  wires:
  Radians to Degrees1/1 -> Bus Creator/2  "theta_dot_degps"
  pm_pi/1(rad_out) -> Radians to Degrees/1
  xP/1 -> Bus Creator/5  "x_POS"
  theta_dot/1 -> Radians to Degrees1/1
  theta/1 -> pm_pi/1(rad_in)
  Radians to Degrees/1 -> Bus Creator/1  "theta_deg"
  Radians to Degrees3/1 -> Bus Creator/4  "phi_dot_degps"
  vP/1 -> Bus Creator/6  "x_VEL"
  pm_pi1/1(rad_out) -> Radians to Degrees2/1
  Radians to Degrees2/1 -> Bus Creator/3  "phi_deg"
  Bus Creator/1 -> Out1/1
  phi/1 -> pm_pi1/1(rad_in)
  phi_dot/1 -> Radians to Degrees3/1

== system bh_model_crank_dynamics/BRAIN_model/INTEGRATE/Subsystem1 ==
  Constant4 : Constant  Value=params.L_1
  Constant5 : Constant  Value=params.L_2
  L1 : Outport
  L2 : Outport  Port=2
  wires:
  Constant5/1 -> L2/1
  Constant4/1 -> L1/1

== system bh_model_crank_dynamics/BRAIN_model/INTEGRATE/Subsystem2 ==
  Constant4 : Constant  Value=params.L_1
  Constant5 : Constant  Value=params.L_2
  L1 : Outport
  L2 : Outport  Port=2
  wires:
  Constant5/1 -> L2/1
  Constant4/1 -> L1/1

== system bh_model_crank_dynamics/SIMSCAPE_MODEL/Subsystem1/Subsystem ==
  ANG : Inport
  AXIS : Inport  Port=2
  Compare To Zero : simulink/Logic and Bit Operations/Compare To Zero  relop=>=  OutDataTypeStr=boolean
  Gain : Gain  Gain=-1
  Selector : Selector  InputPortWidth=3  IndexOptions=Index vector (dialog)  Indices=3  OutputSizes=1
  Switch : Switch  Criteria=u2 > Threshold  SaturateOnIntegerOverflow=off  InputSameDT=off
  ANG_OUT : Outport
  wires:
  AXIS/1 -> Selector/1
  Selector/1 -> Compare To Zero/1
  Switch/1 -> ANG_OUT/1
  ANG/1 -> Gain/1, Switch/1
  Compare To Zero/1 -> Switch/2
  Gain/1 -> Switch/3

== system bh_model_crank_dynamics/SIMSCAPE_MODEL/Subsystem2/Subsystem ==
  ANG : Inport
  AXIS : Inport  Port=2
  Compare To Zero : simulink/Logic and Bit Operations/Compare To Zero  relop=>=  OutDataTypeStr=boolean
  Gain : Gain  Gain=-1
  Selector : Selector  InputPortWidth=3  IndexOptions=Index vector (dialog)  Indices=3  OutputSizes=1
  Switch : Switch  Criteria=u2 > Threshold  SaturateOnIntegerOverflow=off  InputSameDT=off
  ANG_OUT : Outport
  wires:
  AXIS/1 -> Selector/1
  Selector/1 -> Compare To Zero/1
  Switch/1 -> ANG_OUT/1
  ANG/1 -> Gain/1, Switch/1
  Compare To Zero/1 -> Switch/2
  Gain/1 -> Switch/3

== system bh_model_crank_dynamics/SIMSCAPE_MODEL/make_BUS/pm_pi ==
  rad_in : Inport
  Trigonometric Function : Trigonometry  Operator=atan2
  Trigonometric Function1 : Trigonometry
  Trigonometric Function2 : Trigonometry  Operator=cos
  rad_out : Outport
  wires:
  rad_in/1 -> Trigonometric Function2/1, Trigonometric Function1/1
  Trigonometric Function2/1 -> Trigonometric Function/2
  Trigonometric Function1/1 -> Trigonometric Function/1
  Trigonometric Function/1 -> rad_out/1

== system bh_model_crank_dynamics/SIMSCAPE_MODEL/make_BUS/pm_pi1 ==
  rad_in : Inport
  Trigonometric Function : Trigonometry  Operator=atan2
  Trigonometric Function1 : Trigonometry
  Trigonometric Function2 : Trigonometry  Operator=cos
  rad_out : Outport
  wires:
  rad_in/1 -> Trigonometric Function2/1, Trigonometric Function1/1
  Trigonometric Function2/1 -> Trigonometric Function/2
  Trigonometric Function1/1 -> Trigonometric Function/1
  Trigonometric Function/1 -> rad_out/1
